simulink model "Lab2"  (R2022b)
settings: Solver=FixedStepAuto  StartTime=0.0  StopTime=59.25  FixedStep=0.02  RelTol=1e-3
undefined symbols (not defined in the file): unicycle, X, Y
libraries: robotlib x9
settings Model: Creator=Musta  LastModifiedBy=mustacchim
settings OptimizationCC: EnhancedBackFolding=on  PassReuseOutputArgsAs=Individual arguments  ZeroExternalMemoryAtStartup=off  ZeroInternalMemoryAtStartup=off  MaxStackSize=64  OptimizeBlockOrder=speed  DifferentSizesBufferReuse=on  OptimizationCustomize=off  EfficientTunableParamExpr=on
settings DebuggingCC: ParameterTunabilityLossMsg=error
settings HardwareCC: ProdBitPerPointer=32  ProdBitPerSizeT=32  ProdBitPerPtrDiffT=32  ProdLargestAtomicFloat=None  ProdIntDivRoundTo=Undefined  ProdEndianess=Unspecified  ProdWordSize=32  ProdHWDeviceType=Generic->Unspecified (assume 32-bit Generic)
settings SFSimCC: MATLABDynamicMemAlloc=off
settings RTWCC: Description=Embedded Coder  SystemTargetFile=ert.tlc  HardwareBoard=Robot Operating System (ROS)  TLCOptions="-aInlineSetEventsForThisBaseRateFcn=TLC_FALSE -aSuppressMultiTaskScheduler=TLC_FALSE  -aRateBasedStepFcn=0"  TemplateMakefile=ert_default_tmf  Toolchain=Catkin  TargetLang=C++
settings CodeAppCC: ForceParamTrailComments=on  IgnoreCustomStorageClasses=off  OperatorAnnotations=on  SimulinkDataObjDesc=on  SFDataObjDesc=on  InsertBlockDesc=on

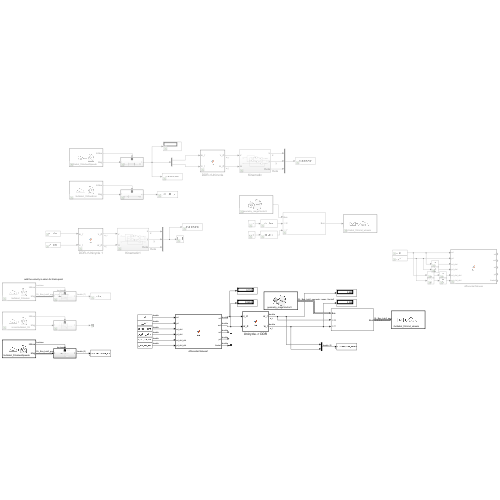
[thumbnail: Simulink's stored preview of the top-level diagram]
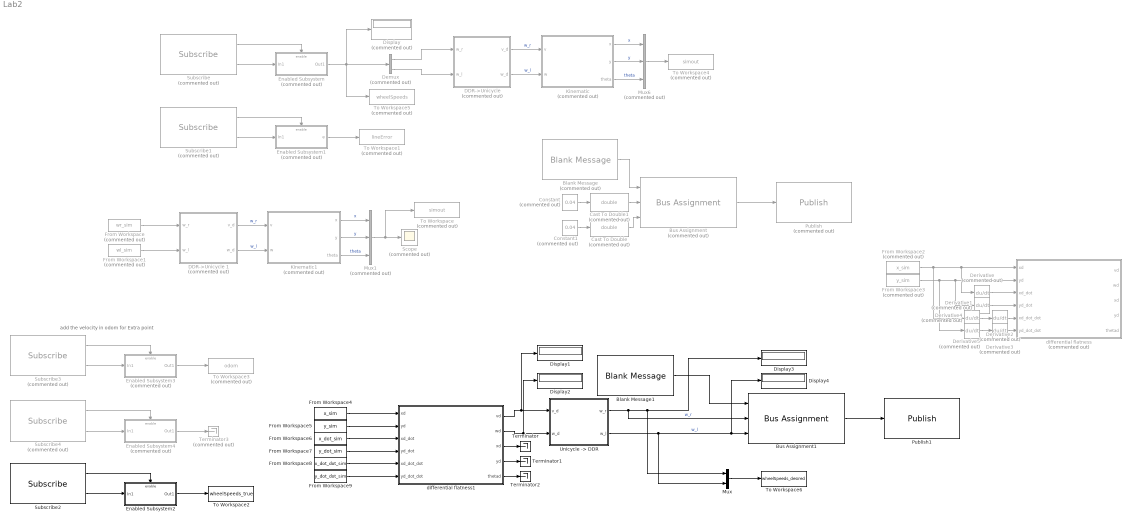
== system Lab2 ==
  note: add the velocity in odom for Extra point
  " DDR->Unicycle " : MATLAB Function  Commented=on  TreatAsAtomicUnit=on
  " DDR->Unicycle 1" : MATLAB Function  Commented=on  TreatAsAtomicUnit=on
  Blank Message : robotlib/Blank Message  Commented=on  messageClass=Message  entityType=geometry_msgs/Vector3  messageType=geometry_msgs/Vector3  SampleTime=0.02  legacyBusStruct=off
      settings: LibrarySourceBlock=roslib/ROS/Blank Message
  Blank Message1 : robotlib/Blank Message  messageClass=Message  entityType=geometry_msgs/Vector3  messageType=geometry_msgs/Vector3  SampleTime=0.02  legacyBusStruct=off
      settings: LibrarySourceBlock=roslib/ROS/Blank Message
  Bus Assignment : BusAssignment  Commented=on  AssignedSignals=X,Y
  Bus Assignment1 : BusAssignment  AssignedSignals=X,Y
  Cast To Double : DataTypeConversion  Commented=on  OutDataTypeStr=double  SaturateOnIntegerOverflow=off  RndMeth=Floor
  Cast To Double1 : DataTypeConversion  Commented=on  OutDataTypeStr=double  SaturateOnIntegerOverflow=off  RndMeth=Floor
  Constant : Constant  Commented=on  Value=0.04
  Constant1 : Constant  Commented=on  Value=0.04
  Demux : Demux  Commented=on  Outputs=2
  Derivative{,1..5} (6 alike) : Derivative  Commented=on
  Display : Display  Commented=on
  Display{1..4} (4 alike) : Display
  Enabled Subsystem : Subsystem  Commented=on  TreatAsAtomicUnit=on
  Enabled Subsystem1 : Subsystem  Commented=on  TreatAsAtomicUnit=on
  Enabled Subsystem2 : Subsystem  TreatAsAtomicUnit=on
  Enabled Subsystem3 : Subsystem  Commented=on  TreatAsAtomicUnit=on
  Enabled Subsystem4 : Subsystem  Commented=on  TreatAsAtomicUnit=on
  From Workspace : FromWorkspace  Commented=on  VariableName=wr_sim
  From Workspace1 : FromWorkspace  Commented=on  VariableName=wl_sim
  From Workspace2 : FromWorkspace  Commented=on  VariableName=x_sim
  From Workspace3 : FromWorkspace  Commented=on  VariableName=y_sim
  From Workspace4 : FromWorkspace  VariableName=x_sim
  From Workspace5 : FromWorkspace  VariableName=y_sim
  From Workspace6 : FromWorkspace  VariableName=x_dot_sim
  From Workspace7 : FromWorkspace  VariableName=y_dot_sim
  From Workspace8 : FromWorkspace  VariableName=x_dot_dot_sim
  From Workspace9 : FromWorkspace  VariableName=y_dot_dot_sim
  Kinematic : Subsystem  Commented=on
  Kinematic1 : Subsystem  Commented=on
  Mux : Mux  Inputs=2
  Mux1 : Mux  Commented=on  Inputs=3
  Mux6 : Mux  Commented=on  Inputs=3
  Publish : robotlib/Publish  Commented=on  topicSource=Select from ROS network  topic=/turtlebot_03/cmd_wheels  messageType=geometry_msgs/Vector3  legacyBusStruct=off  messageQueueLength=1
      settings: LibrarySourceBlock=roslib/ROS/Publish
  Publish1 : robotlib/Publish  topicSource=Select from ROS network  topic=/turtlebot_03/cmd_wheels  messageType=geometry_msgs/Vector3  legacyBusStruct=off  messageQueueLength=1
      settings: LibrarySourceBlock=roslib/ROS/Publish
  Scope : Scope  Commented=on
  Subscribe : robotlib/Subscribe  Commented=on  topicSource=Select from ROS network  topic=/turtlebot_03/wheelSpeeds  messageType=geometry_msgs/Vector3  SampleTime=0.02  legacyBusStruct=off  messageQueueLength=1
      settings: LibrarySourceBlock=roslib/ROS/Subscribe
  Subscribe1 : robotlib/Subscribe  Commented=on  topicSource=Select from ROS network  topic=/turtlebot_03/lineError  messageType=std_msgs/Float32  SampleTime=0.10  legacyBusStruct=off  messageQueueLength=1
      settings: LibrarySourceBlock=roslib/ROS/Subscribe
  Subscribe2 : robotlib/Subscribe  topicSource=Select from ROS network  topic=/turtlebot_03/wheelSpeeds  messageType=geometry_msgs/Vector3  SampleTime=0.02  legacyBusStruct=off  messageQueueLength=1
      settings: LibrarySourceBlock=roslib/ROS/Subscribe
  Subscribe3 : robotlib/Subscribe  Commented=on  topicSource=Select from ROS network  topic=/turtlebot_03/odom  messageType=nav_msgs/Odometry  SampleTime=0.02  legacyBusStruct=off  messageQueueLength=1
      settings: LibrarySourceBlock=roslib/ROS/Subscribe
  Subscribe4 : robotlib/Subscribe  Commented=on  topicSource=Select from ROS network  topic=/vicon/turtlebot_03  messageType=vicon/Subject  SampleTime=0.02  legacyBusStruct=off  messageQueueLength=1
      settings: LibrarySourceBlock=roslib/ROS/Subscribe
  Terminator : Terminator
  Terminator1 : Terminator
  Terminator2 : Terminator
  Terminator3 : Terminator  Commented=on
  To Workspace : ToWorkspace  Commented=on  VariableName=simout  SaveFormat=Structure With Time  SampleTime=-1
  To Workspace1 : ToWorkspace  Commented=on  VariableName=lineError  SaveFormat=Structure With Time  SampleTime=-1
  To Workspace2 : ToWorkspace  VariableName=wheelSpeeds_true  SaveFormat=Structure With Time  SampleTime=-1
  To Workspace3 : ToWorkspace  Commented=on  VariableName=odom  SaveFormat=Structure With Time  SampleTime=-1
  To Workspace4 : ToWorkspace  Commented=on  VariableName=simout  SaveFormat=Structure With Time  SampleTime=-1
  To Workspace5 : ToWorkspace  Commented=on  VariableName=wheelSpeeds  SaveFormat=Structure With Time  SampleTime=-1
  To Workspace6 : ToWorkspace  VariableName=wheelSpeeds_desired  SaveFormat=Structure With Time  SampleTime=-1
  "Unicycle -> DDR" : MATLAB Function  TreatAsAtomicUnit=on
  differential flatness : MATLAB Function  Commented=on  TreatAsAtomicUnit=on
  differential flatness1 : MATLAB Function  TreatAsAtomicUnit=on
  wires:
  " DDR->Unicycle "/1(v_d) -> Kinematic/1(v)  "w_r"
  " DDR->Unicycle "/2(w_d) -> Kinematic/2(w)  "w_l"
  Kinematic/1(x) -> Mux6/1  "x"
  Kinematic/3(theta) -> Mux6/3  "theta"
  Kinematic/2(y) -> Mux6/2  "y"
  Mux6/1 -> To Workspace4/1
  Subscribe/1 -> Enabled Subsystem/Enable
  Enabled Subsystem/1(Out1) -> To Workspace5/1, Demux/1, Display/1
  Subscribe/2 -> Enabled Subsystem/1(In1)
  Demux/1 -> " DDR->Unicycle "/1(w_r)
  Demux/2 -> " DDR->Unicycle "/2(w_l)
  Subscribe1/2 -> Enabled Subsystem1/1(In1)
  Subscribe1/1 -> Enabled Subsystem1/Enable
  Enabled Subsystem1/1(e) -> To Workspace1/1
  Bus Assignment/1 -> Publish/1
  Blank Message/1 -> Bus Assignment/1
  Mux1/1 -> To Workspace/1, Scope/1
  Kinematic1/3(theta) -> Mux1/3  "theta"
  " DDR->Unicycle 1"/1(v_d) -> Kinematic1/1(v)  "w_r"
  Kinematic1/2(y) -> Mux1/2  "y"
  " DDR->Unicycle 1"/2(w_d) -> Kinematic1/2(w)  "w_l"
  Kinematic1/1(x) -> Mux1/1  "x"
  From Workspace/1 -> " DDR->Unicycle 1"/1(w_r)
  From Workspace1/1 -> " DDR->Unicycle 1"/2(w_l)
  Blank Message1/1 -> Bus Assignment1/1
  Bus Assignment1/1 -> Publish1/1
  differential flatness1/1(vd) -> Display1/1, "Unicycle -> DDR"/1(v_d)
  differential flatness1/2(wd) -> Display2/1, "Unicycle -> DDR"/2(w_d)
  "Unicycle -> DDR"/1(w_r) -> Bus Assignment1/2, Mux/1, Display3/1  "w_r"
  "Unicycle -> DDR"/2(w_l) -> Mux/2, Bus Assignment1/3, Display4/1  "w_l"
  differential flatness1/3(xd) -> Terminator/1
  differential flatness1/4(yd) -> Terminator1/1
  differential flatness1/5(thetad) -> Terminator2/1
  Subscribe2/1 -> Enabled Subsystem2/Enable
  Subscribe2/2 -> Enabled Subsystem2/1(In1)
  Enabled Subsystem2/1(Out1) -> To Workspace2/1
  Enabled Subsystem3/1(Out1) -> To Workspace3/1
  Subscribe3/2 -> Enabled Subsystem3/1(In1)
  Subscribe3/1 -> Enabled Subsystem3/Enable
  Mux/1 -> To Workspace6/1
  From Workspace4/1 -> differential flatness1/1("xd ")
  From Workspace5/1 -> differential flatness1/2("yd ")
  From Workspace9/1 -> differential flatness1/6(yd_dot_dot)
  From Workspace8/1 -> differential flatness1/5(xd_dot_dot)
  From Workspace7/1 -> differential flatness1/4(yd_dot)
  From Workspace6/1 -> differential flatness1/3(xd_dot)
  Cast To Double/1 -> Bus Assignment/3
  Constant1/1 -> Cast To Double/1
  Cast To Double1/1 -> Bus Assignment/2
  Constant/1 -> Cast To Double1/1
  Derivative/1 -> differential flatness/3(xd_dot)
  Derivative1/1 -> differential flatness/4(yd_dot)
  Derivative5/1 -> Derivative3/1
  Derivative4/1 -> Derivative2/1
  Derivative3/1 -> differential flatness/6(yd_dot_dot)
  Derivative2/1 -> differential flatness/5(xd_dot_dot)
  From Workspace2/1 -> Derivative4/1, Derivative/1, differential flatness/1("xd ")
  From Workspace3/1 -> Derivative5/1, Derivative1/1, differential flatness/2("yd ")
  Subscribe4/1 -> Enabled Subsystem4/Enable
  Enabled Subsystem4/1(Out1) -> Terminator3/1
  Subscribe4/2 -> Enabled Subsystem4/1(In1)

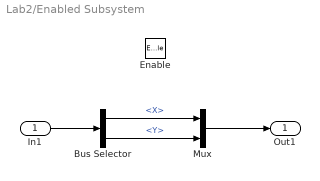
== system Lab2/Enabled Subsystem ==
  In1 : Inport
  Enable : EnablePort
  Bus Selector : BusSelector  OutputSignals=X,Y
  Mux : Mux  Inputs=2
  Out1 : Outport
  wires:
  Mux/1 -> Out1/1
  Bus Selector/1 -> Mux/1  "<X>"
  Bus Selector/2 -> Mux/2  "<Y>"
  In1/1 -> Bus Selector/1

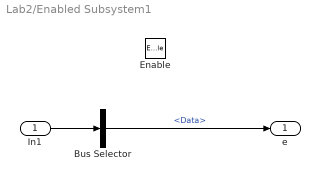
== system Lab2/Enabled Subsystem1 ==
  In1 : Inport
  Enable : EnablePort
  Bus Selector : BusSelector  OutputSignals=Data
  e : Outport
  wires:
  In1/1 -> Bus Selector/1
  Bus Selector/1 -> e/1  "<Data>"

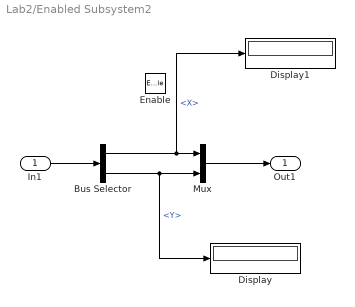
== system Lab2/Enabled Subsystem2 ==
  In1 : Inport
  Enable : EnablePort
  Bus Selector : BusSelector  OutputSignals=X,Y
  Display : Display
  Display1 : Display
  Mux : Mux  Inputs=2
  Out1 : Outport
  wires:
  Mux/1 -> Out1/1
  Bus Selector/1 -> Display1/1, Mux/1  "<X>"
  Bus Selector/2 -> Display/1, Mux/2  "<Y>"
  In1/1 -> Bus Selector/1

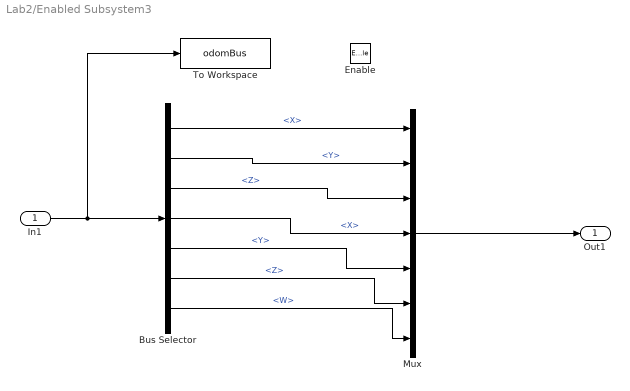
== system Lab2/Enabled Subsystem3 ==
  In1 : Inport
  Enable : EnablePort
  Bus Selector : BusSelector  OutputSignals=Pose.Pose.Position.X,Pose.Pose.Position.Y,Pose.Pose.Position.Z,Pose.Pose.Orientation.X,Pose.Pose.Orientation.Y,Pose.Pose.Orientation.Z,Pose.Pose.Orientation.W
  Mux : Mux  Inputs=7
  To Workspace : ToWorkspace  VariableName=odomBus  SaveFormat=Timeseries  SampleTime=-1
  Out1 : Outport
  wires:
  Mux/1 -> Out1/1
  Bus Selector/1 -> Mux/1  "<X>"
  Bus Selector/2 -> Mux/2  "<Y>"
  In1/1 -> To Workspace/1, Bus Selector/1
  Bus Selector/3 -> Mux/3  "<Z>"
  Bus Selector/4 -> Mux/4  "<X>"
  Bus Selector/5 -> Mux/5  "<Y>"
  Bus Selector/6 -> Mux/6  "<Z>"
  Bus Selector/7 -> Mux/7  "<W>"

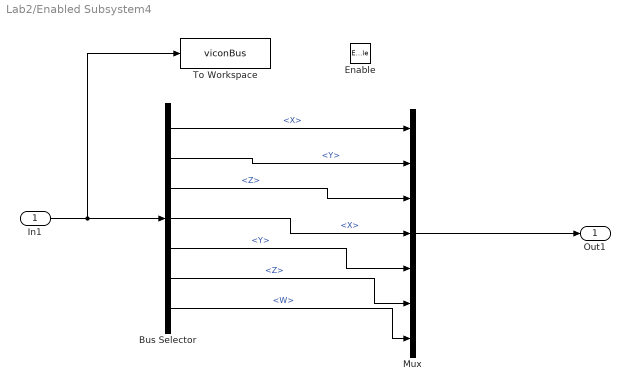
== system Lab2/Enabled Subsystem4 ==
  In1 : Inport
  Enable : EnablePort
  Bus Selector : BusSelector  OutputSignals=Pose.Pose.Position.X,Pose.Pose.Position.Y,Pose.Pose.Position.Z,Pose.Pose.Orientation.X,Pose.Pose.Orientation.Y,Pose.Pose.Orientation.Z,Pose.Pose.Orientation.W
  Mux : Mux  Inputs=7
  To Workspace : ToWorkspace  VariableName=viconBus  SaveFormat=Timeseries  SampleTime=-1
  Out1 : Outport
  wires:
  Mux/1 -> Out1/1
  Bus Selector/1 -> Mux/1  "<X>"
  Bus Selector/2 -> Mux/2  "<Y>"
  In1/1 -> To Workspace/1, Bus Selector/1
  Bus Selector/3 -> Mux/3  "<Z>"
  Bus Selector/4 -> Mux/4  "<X>"
  Bus Selector/5 -> Mux/5  "<Y>"
  Bus Selector/6 -> Mux/6  "<Z>"
  Bus Selector/7 -> Mux/7  "<W>"

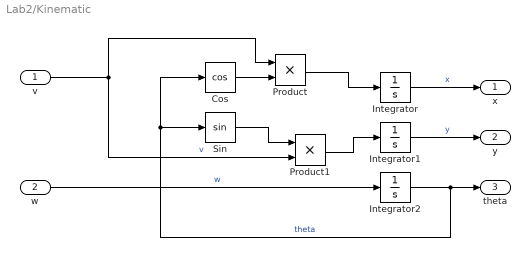
== system Lab2/Kinematic ==
  v : Inport
  w : Inport  Port=2
  Cos : Trigonometry  Operator=cos
  Integrator : Integrator  InitialCondition=unicycle.ic.x
  Integrator1 : Integrator  InitialCondition=unicycle.ic.y
  Integrator2 : Integrator  InitialCondition=unicycle.ic.theta
  Product : Product
  Product1 : Product
  Sin : Trigonometry
  x : Outport
  y : Outport  Port=2
  theta : Outport  Port=3
  wires:
  w/1 -> Integrator2/1  "w"
  Product/1 -> Integrator/1
  v/1 -> Product/1, Product1/2  "v"
  Cos/1 -> Product/2
  Integrator1/1 -> y/1  "y"
  Integrator/1 -> x/1  "x"
  Integrator2/1 -> Cos/1, Sin/1, theta/1  "theta"
  Product1/1 -> Integrator1/1
  Sin/1 -> Product1/1

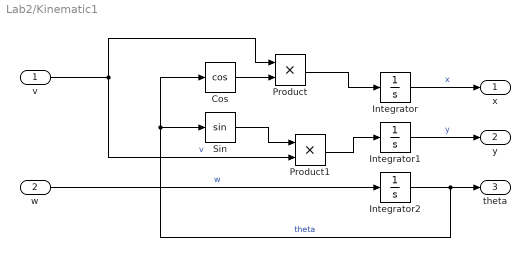
== system Lab2/Kinematic1 ==
  v : Inport
  w : Inport  Port=2
  Cos : Trigonometry  Operator=cos
  Integrator : Integrator  InitialCondition=unicycle.ic.x
  Integrator1 : Integrator  InitialCondition=unicycle.ic.y
  Integrator2 : Integrator  InitialCondition=unicycle.ic.theta
  Product : Product
  Product1 : Product
  Sin : Trigonometry
  x : Outport
  y : Outport  Port=2
  theta : Outport  Port=3
  wires:
  w/1 -> Integrator2/1  "w"
  Product/1 -> Integrator/1
  v/1 -> Product/1, Product1/2  "v"
  Cos/1 -> Product/2
  Integrator1/1 -> y/1  "y"
  Integrator/1 -> x/1  "x"
  Integrator2/1 -> Cos/1, Sin/1, theta/1  "theta"
  Product1/1 -> Integrator1/1
  Sin/1 -> Product1/1

== matlab function Lab2/ DDR->Unicycle  ==
  data: w_r input; v_d output; w_l input; w_d output
function [v_d, w_d] = fcn( w_r, w_l)

    %#codegen
    coder.extrinsic('evalin')
    d = 0;                  % Needed in order to set variable class correctly
    r = 0;                  % Needed in order to set variable class correctly
    d = evalin('base','unicycle.d'); % Read value from workspace
    r = evalin('base','unicycle.r'); % Read value from workspace

    v_d = r*( w_r + w_l)/2;
    w_d = r*( w_r - w_l)/d;
    

end

== matlab function Lab2/ DDR->Unicycle 1 ==
  data: w_r input; v_d output; w_l input; w_d output
function [v_d, w_d] = fcn(w_r, w_l)

    %#codegen
    coder.extrinsic('evalin')
    d = 0;                  % Needed in order to set variable class correctly
    r = 0;                  % Needed in order to set variable class correctly
    d = evalin('base','unicycle.d'); % Read value from workspace
    r = evalin('base','unicycle.r'); % Read value from workspace

    v_d = r*(w_r + w_l)/2;
    w_d = r*(w_r - w_l)/d;
    

end

== matlab function Lab2/differential flatness ==
  data: xd input; vd output; yd input; xd_dot input; yd_dot input; xd_dot_dot input; yd_dot_dot input; wd output; xd output; yd output; thetad output
function [vd, wd, xd, yd, thetad] = fcn(xd, yd, xd_dot, yd_dot, xd_dot_dot, yd_dot_dot)
    
    vd = sqrt(xd_dot.^2 + yd_dot.^2);
    wd = (xd_dot.*yd_dot_dot - xd_dot_dot.*yd_dot) / (xd_dot.^2 + yd_dot.^2);
    % thetad = atan2(yd_dot, xd_dot);
    thetad = mod(atan2(yd_dot,xd_dot), 2*pi);

    xd = xd;
    yd = yd;

end

== matlab function Lab2/differential flatness1 ==
  data: xd input; vd output; yd input; xd_dot input; yd_dot input; xd_dot_dot input; yd_dot_dot input; wd output; xd output; yd output; thetad output
function [vd, wd, xd, yd, thetad] = fcn(xd, yd, xd_dot, yd_dot, xd_dot_dot, yd_dot_dot)
    
    vd = sqrt(xd_dot.^2 + yd_dot.^2);
    wd = (xd_dot.*yd_dot_dot - xd_dot_dot.*yd_dot) / (xd_dot.^2 + yd_dot.^2);
    % thetad = atan2(yd_dot, xd_dot);
    thetad = mod(atan2(yd_dot,xd_dot), 2*pi);

    xd = xd;
    yd = yd;

end

== matlab function Lab2/Unicycle -> DDR ==
  data: v_d input; w_r output; w_d input; w_l output
function [w_r, w_l] = fcn(v_d, w_d)

    %#codegen
    coder.extrinsic('evalin')
    d = 0;                  % Needed in order to set variable class correctly
    r = 0;                  % Needed in order to set variable class correctly
    d = evalin('base','unicycle.d'); % Read value from workspace
    r = evalin('base','unicycle.r'); % Read value from workspace

    w_r = ((2 * v_d) + (w_d * d)) / (2 * r);
    w_l = ((2 * v_d) - (w_d * d)) / (2 * r);

end
